simulink model "simSystemId"  (R2020a)
settings: Solver=ode4  StartTime=1.25e-4  StopTime=3.75  FixedStep=1.25e-4  RelTol=1e-3
values from neighbouring files (symbols this model uses):
  numS = [zeros(1, delayS),numS]    [identificationDelaytest.m]    (also in systemIddemo.m)
undefined symbols (not defined in the file or in its folder): denS
libraries: simulink x1
settings Model: Creator=胡子瀚  LastModifiedBy=胡子瀚

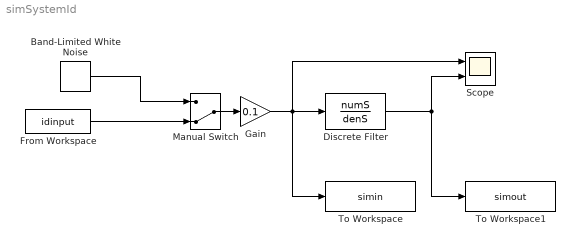
== system simSystemId ==
  Band-Limited White Noise : simulink/Sources/Band-Limited White Noise  Cov=[0.1]  Ts=1.25e-4  seed=[23341]
  Discrete Filter : DiscreteFilter  Numerator=numS  Denominator=denS
  From Workspace : FromWorkspace  VariableName=idinput
  Gain : Gain  Gain=0.1
  Manual Switch : ManualSwitch  CurrentSetting=0
  Scope : Scope  NumInputPorts=2
  To Workspace : ToWorkspace  VariableName=simin  SampleTime=-1
  To Workspace1 : ToWorkspace  VariableName=simout  SampleTime=-1
  wires:
  From Workspace/1 -> Manual Switch/2
  Discrete Filter/1 -> To Workspace1/1, Scope/2
  Gain/1 -> Scope/1, Discrete Filter/1, To Workspace/1
  Manual Switch/1 -> Gain/1
  Band-Limited White Noise/1 -> Manual Switch/1
